simulink model "Copy_of_rigid_body_dynamics"  (R2024b)
settings: Solver=VariableStepAuto  StartTime=0.0  StopTime=50  FixedStep=0.001  RelTol=1e-3
values from neighbouring files (symbols this model uses):
  q_home = [0 15 -130 0 55 90]'*pi/180    [control_dosrobots.m]    (also in rigid_body_dynamics.m = [0 15 -130 0 55 90]' * pi / 180; rigid_body_dynamics_init.m = [0 15 -130 0 55 90]' * pi / 180; trying.m = [0 15 -130 0 55 90]' * pi / 180)
undefined symbols (not defined in the file or in its folder): K_D, K_P
libraries: robotmaniplib x5
settings Model: Creator=spenu  LastModifiedBy=spenu

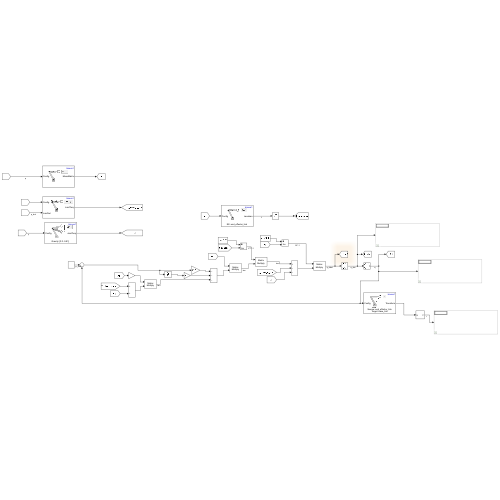
[thumbnail: Simulink's stored preview of the top-level diagram]
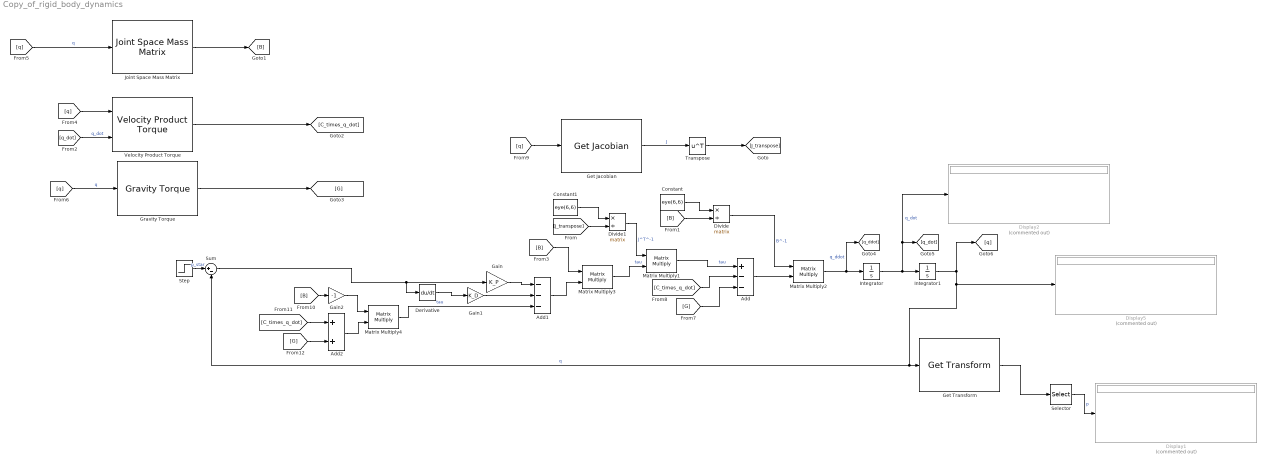
== system Copy_of_rigid_body_dynamics ==
  Add : Sum  Inputs=+--
  Add1 : Sum  Inputs=---
  Add2 : Sum
  Constant : Constant  Value=eye(6,6)
  Constant1 : Constant  Value=eye(6,6)
  Derivative : Derivative
  Display1 : Display  Commented=on
  Display2 : Display  Commented=on
  Display5 : Display  Commented=on
  Divide : Product  Inputs=*/  Multiplication=Matrix(*)
  Divide1 : Product  Inputs=*/  Multiplication=Matrix(*)
  Gain : Gain  Gain=K_P
  Gain1 : Gain  Gain=K_D
  Gain2 : Gain  Gain=-1
  Get Jacobian : robotmaniplib/Get Jacobian  RigidBodyTree=kinova1  EndEffector=end_effector_link  SimulateUsing=Interpreted execution
  Get Transform : robotmaniplib/Get Transform  RigidBodyTree=kinova1  SourceBody=end_effector_link  TargetBody=base_link  SimulateUsing=Interpreted execution
  Gravity Torque : robotmaniplib/Gravity Torque  RigidBodyTree=kinova1  SimulateUsing=Interpreted execution
  Integrator : Integrator  WrapState=on  WrappedStateUpperValue=2*pi  WrappedStateLowerValue=-2*pi
  Integrator1 : Integrator  WrapState=on
  Joint Space Mass Matrix : robotmaniplib/Joint Space Mass Matrix  RigidBodyTree=kinova1  SimulateUsing=Interpreted execution
  Matrix Multiply{1..4} (4 alike) : Product  Multiplication=Matrix(*)
  Selector : Selector  NumberOfDimensions=2  InputPortWidth=3  IndexOptions=Index vector (dialog),Starting index (dialog)  Indices=[1:3],4  OutputSizes=1,1  RuntimeRangeChecks=on
  Step : Step  Time=0.5  Before=q_home  After=q_home  SampleTime=0
  Sum : Sum  Inputs=|+-
  Transpose : Math  Operator=transpose
  Velocity Product Torque : robotmaniplib/Velocity Product Torque  RigidBodyTree=kinova1  SimulateUsing=Interpreted execution
  wires:
  Joint Space Mass Matrix/1 -> [B]
  [q] -> Joint Space Mass Matrix/1  "q"
  [q_dot] -> Velocity Product Torque/2  "q_dot"
  [q] -> Velocity Product Torque/1
  [q] -> Gravity Torque/1  "q"
  Velocity Product Torque/1 -> [C_times_q_dot]
  Gravity Torque/1 -> [G]
  Selector/1 -> Display1/1  "p"
  Get Jacobian/1 -> Transpose/1  "J"
  Transpose/1 -> [J_transpose]
  Matrix Multiply1/1 -> Add/1  "tau"
  Constant/1 -> Divide/1
  [B] -> Divide/2
  Divide/1 -> Matrix Multiply2/1  "B^-1"
  [G] -> Add/3
  [C_times_q_dot] -> Add/2
  Add/1 -> Matrix Multiply2/2
  Matrix Multiply2/1 -> [q_ddot], Integrator/1  "q_ddot"
  Integrator/1 -> Display2/1, [q_dot], Integrator1/1  "q_dot"
  Integrator1/1 -> [q], Display5/1, Sum/2, Get Transform/1  "q"
  Get Transform/1 -> Selector/1
  [q] -> Get Jacobian/1
  [J_transpose] -> Divide1/2
  Constant1/1 -> Divide1/1
  Divide1/1 -> Matrix Multiply1/1  "J^T^-1"
  Matrix Multiply3/1 -> Matrix Multiply1/2  "tau"
  [B] -> Matrix Multiply3/1
  Add1/1 -> Matrix Multiply3/2
  Gain/1 -> Add1/1
  Gain1/1 -> Add1/2
  [B] -> Gain2/1
  Gain2/1 -> Matrix Multiply4/1
  Matrix Multiply4/1 -> Add1/3  "tau"
  [C_times_q_dot] -> Add2/1
  Add2/1 -> Matrix Multiply4/2
  [G] -> Add2/2
  Step/1 -> Sum/1  "p_star"
  Sum/1 -> Derivative/1, Gain/1
  Derivative/1 -> Gain1/1
